simulink model "SControle"  (R2014b)
settings: Solver=ode45  StartTime=0.0  StopTime=50.0  RelTol=1e-3
libraries: simulink x2
settings Model: Creator=highamj  LastModifiedBy=highamj

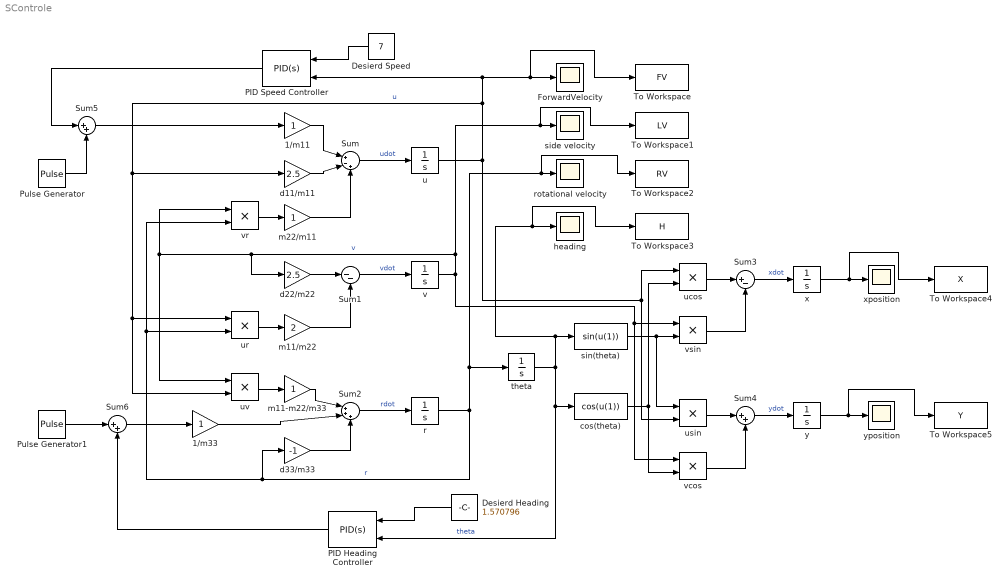
== system SControle ==
  1/m11 : Gain
  1/m33 : Gain
  Desierd Heading : Constant  Value=1.570796
  Desierd Speed : Constant  Value=7
  ForwardVelocity : Scope
      settings: YMin=500000  YMax=1.5e+06  SaveName=ScopeData3
  PID Heading Controller : simulink/Continuous/PID Controller (2DOF)  Controller=PID  TimeDomain=Continuous-time  SampleTime=-1  IntegratorMethod=Forward Euler  FilterMethod=Forward Euler  Form=Parallel  P=5.96375779922345  I=0.127939709833734  D=1.41156755886535  N=5.23154506794489  b=1  c=1  InitialConditionSource=internal  InitialConditionForIntegrator=0  InitialConditionForFilter=0  ExternalReset=none  LimitOutput=off  UpperSaturationLimit=inf  LowerSaturationLimit=-inf  LinearizeAsGain=on  AntiWindupMode=none  Kb=1  TrackingMode=off  Kt=1  PParamMin=[]  PParamMax=[]  IParamMin=[]  IParamMax=[]  DParamMin=[]  DParamMax=[]  NParamMin=[]  NParamMax=[]  bParamMin=[]  bParamMax=[]  cParamMin=[]  cParamMax=[]  KbParamMin=[]  KbParamMax=[]  KtParamMin=[]  KtParamMax=[]  POutMin=[]  POutMax=[]  IOutMin=[]  IOutMax=[]  DOutMin=[]  DOutMax=[]  NOutMin=[]  NOutMax=[]  bOutMin=[]  bOutMax=[]  cOutMin=[]  cOutMax=[]  KbOutMin=[]  KbOutMax=[]  KtOutMin=[]  KtOutMax=[]  IntegratorOutMin=[]  IntegratorOutMax=[]  FilterOutMin=[]  FilterOutMax=[]  SumOutMin=[]  SumOutMax=[]  Sum1OutMin=[]  Sum1OutMax=[]  Sum2OutMin=[]  Sum2OutMax=[]  Sum3OutMin=[]  Sum3OutMax=[]  SumI1OutMin=[]  SumI1OutMax=[]  SumI2OutMin=[]  SumI2OutMax=[]  SumI3OutMin=[]  SumI3OutMax=[]  SumDOutMin=[]  SumDOutMax=[]  SaturationOutMin=[]  SaturationOutMax=[]  IntegratorContinuousStateAttributes=''  IntegratorStateMustResolveToSignalObject=off  IntegratorRTWStateStorageClass=Auto  FilterContinuousStateAttributes=''  FilterStateMustResolveToSignalObject=off  FilterRTWStateStorageClass=Auto  DifferentiatorICPrevScaledInput=0  DifferentiatorOutMin=[]  DifferentiatorOutMax=[]  UseFilter=on
  PID Speed Controller : simulink/Continuous/PID Controller (2DOF)  Controller=PID  TimeDomain=Continuous-time  SampleTime=-1  IntegratorMethod=Forward Euler  FilterMethod=Forward Euler  Form=Parallel  P=0  I=4.52260515354749  D=0  N=100  b=1  c=1  InitialConditionSource=internal  InitialConditionForIntegrator=0  InitialConditionForFilter=0  ExternalReset=none  LimitOutput=off  UpperSaturationLimit=inf  LowerSaturationLimit=-inf  LinearizeAsGain=on  AntiWindupMode=none  Kb=1  TrackingMode=off  Kt=1  PParamMin=[]  PParamMax=[]  IParamMin=[]  IParamMax=[]  DParamMin=[]  DParamMax=[]  NParamMin=[]  NParamMax=[]  bParamMin=[]  bParamMax=[]  cParamMin=[]  cParamMax=[]  KbParamMin=[]  KbParamMax=[]  KtParamMin=[]  KtParamMax=[]  POutMin=[]  POutMax=[]  IOutMin=[]  IOutMax=[]  DOutMin=[]  DOutMax=[]  NOutMin=[]  NOutMax=[]  bOutMin=[]  bOutMax=[]  cOutMin=[]  cOutMax=[]  KbOutMin=[]  KbOutMax=[]  KtOutMin=[]  KtOutMax=[]  IntegratorOutMin=[]  IntegratorOutMax=[]  FilterOutMin=[]  FilterOutMax=[]  SumOutMin=[]  SumOutMax=[]  Sum1OutMin=[]  Sum1OutMax=[]  Sum2OutMin=[]  Sum2OutMax=[]  Sum3OutMin=[]  Sum3OutMax=[]  SumI1OutMin=[]  SumI1OutMax=[]  SumI2OutMin=[]  SumI2OutMax=[]  SumI3OutMin=[]  SumI3OutMax=[]  SumDOutMin=[]  SumDOutMax=[]  SaturationOutMin=[]  SaturationOutMax=[]  IntegratorContinuousStateAttributes=''  IntegratorStateMustResolveToSignalObject=off  IntegratorRTWStateStorageClass=Auto  FilterContinuousStateAttributes=''  FilterStateMustResolveToSignalObject=off  FilterRTWStateStorageClass=Auto  DifferentiatorICPrevScaledInput=0  DifferentiatorOutMin=[]  DifferentiatorOutMax=[]  UseFilter=on
  Pulse Generator : DiscretePulseGenerator  PulseType=Time based  Amplitude=5  Period=5  PulseWidth=10
  Pulse Generator1 : DiscretePulseGenerator  PulseType=Time based  Amplitude=-1.570796  Period=25  PulseWidth=10
  Sum : Sum  Inputs=|+-+
  Sum1 : Sum  Inputs=|--
  Sum2 : Sum  Inputs=|+++
  Sum3 : Sum  Inputs=|+-
  Sum4 : Sum  Inputs=|++
  Sum5 : Sum  Inputs=|++
  Sum6 : Sum  Inputs=|++
  To Workspace : ToWorkspace  VariableName=FV  SaveFormat=Timeseries  SampleTime=-1
  To Workspace1 : ToWorkspace  VariableName=LV  SaveFormat=Timeseries  SampleTime=-1
  To Workspace2 : ToWorkspace  VariableName=RV  SaveFormat=Timeseries  SampleTime=-1
  To Workspace3 : ToWorkspace  VariableName=H  SaveFormat=Timeseries  SampleTime=-1
  To Workspace4 : ToWorkspace  VariableName=X  SaveFormat=Timeseries  SampleTime=-1
  To Workspace5 : ToWorkspace  VariableName=Y  SaveFormat=Timeseries  SampleTime=-1
  cos(theta) : Fcn  Expr=cos(u(1))
  d11/m11 : Gain  Gain=2.5
  d22/m22 : Gain  Gain=2.5
  d33/m33 : Gain  Gain=-1
  heading : Scope
      settings: YMin=-140000  YMax=-70000  SaveName=ScopeData2  SampleInput=on
  m11-m22/m33 : Gain
  m11/m22 : Gain  Gain=2
  m22/m11 : Gain
  r : Integrator
  rotational velocity : Scope
      settings: SaveName=ScopeData4
  side velocity : Scope
      settings: SaveName=ScopeData5
  sin(theta) : Fcn  Expr=sin(u(1))
  theta : Integrator  InitialCondition=-0.785398
  u : Integrator
  ucos : Product
  ur : Product
  usin : Product
  uv : Product
  v : Integrator
  vcos : Product
  vr : Product
  vsin : Product
  x : Integrator
  xposition : Scope
  y : Integrator
  yposition : Scope
  wires:
  vr/1 -> m22/m11/1
  v/1 -> To Workspace1/1, side velocity/1, vr/1, uv/1, d22/m22/1, vsin/1, vcos/1  "v"
  r/1 -> To Workspace2/1, rotational velocity/1, theta/1, vr/2, ur/2, d33/m33/1  "r"
  Sum/1 -> u/1  "udot"
  Sum1/1 -> v/1  "vdot"
  Sum2/1 -> r/1  "rdot"
  m22/m11/1 -> Sum/3
  u/1 -> PID Speed Controller/2, To Workspace/1, ForwardVelocity/1, uv/2, ur/1, d11/m11/1, ucos/1, usin/2  "u"
  d11/m11/1 -> Sum/2
  1/m11/1 -> Sum/1
  ur/1 -> m11/m22/1
  m11/m22/1 -> Sum1/2
  d22/m22/1 -> Sum1/1
  d33/m33/1 -> Sum2/3
  m11-m22/m33/1 -> Sum2/1
  uv/1 -> m11-m22/m33/1
  theta/1 -> To Workspace3/1, heading/1, sin(theta)/1, PID Heading Controller/2, cos(theta)/1  "theta"
  Sum4/1 -> y/1  "ydot"
  Sum3/1 -> x/1  "xdot"
  sin(theta)/1 -> vsin/2, usin/1
  cos(theta)/1 -> vcos/2, ucos/2
  ucos/1 -> Sum3/1
  vsin/1 -> Sum3/2
  usin/1 -> Sum4/1
  vcos/1 -> Sum4/2
  x/1 -> To Workspace4/1, xposition/1
  y/1 -> To Workspace5/1, yposition/1
  1/m33/1 -> Sum2/2
  Desierd Heading/1 -> PID Heading Controller/1
  Desierd Speed/1 -> PID Speed Controller/1
  Sum5/1 -> 1/m11/1
  Pulse Generator/1 -> Sum5/2
  PID Speed Controller/1 -> Sum5/1
  Sum6/1 -> 1/m33/1
  Pulse Generator1/1 -> Sum6/1
  PID Heading Controller/1 -> Sum6/2
